simulink model "FOC_algorithm_simulation"  (R2018b)
settings: Solver=VariableStepAuto  StartTime=0.0  StopTime=5  RelTol=1e-3
libraries: simulink x1
settings Model: Creator=杨天山  LastModifiedBy=杨天山

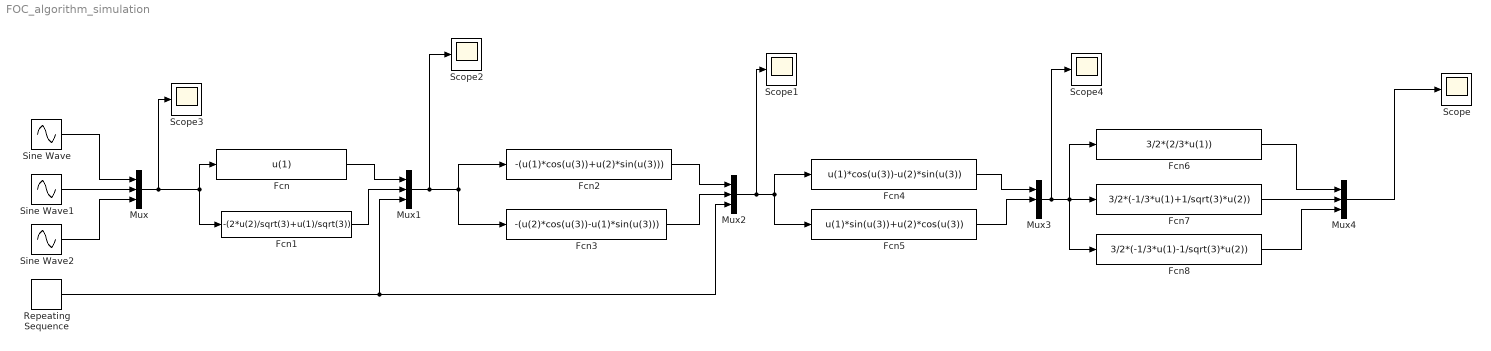
== system FOC_algorithm_simulation ==
  Fcn : Fcn  Expr=u(1)
  Fcn1 : Fcn  Expr=-(2*u(2)/sqrt(3)+u(1)/sqrt(3))
  Fcn2 : Fcn  Expr=-(u(1)*cos(u(3))+u(2)*sin(u(3)))
  Fcn3 : Fcn  Expr=-(u(2)*cos(u(3))-u(1)*sin(u(3)))
  Fcn4 : Fcn  Expr=u(1)*cos(u(3))-u(2)*sin(u(3))
  Fcn5 : Fcn  Expr=u(1)*sin(u(3))+u(2)*cos(u(3))
  Fcn6 : Fcn  Expr=3/2*(2/3*u(1))
  Fcn7 : Fcn  Expr=3/2*(-1/3*u(1)+1/sqrt(3)*u(2))
  Fcn8 : Fcn  Expr=3/2*(-1/3*u(1)-1/sqrt(3)*u(2))
  Mux{,1..4} (5 alike) : Mux  Inputs=3
  Repeating Sequence : simulink/Sources/Repeating Sequence  rep_seq_t=[0 0.1]  rep_seq_y=[0 2*pi]
  Scope{,1..4} (5 alike) : Scope
  Sine Wave : Sin  Frequency=20*pi  SampleTime=0
  Sine Wave1 : Sin  Frequency=20*pi  Phase=2*pi/3  SampleTime=0
  Sine Wave2 : Sin  Frequency=20*pi  Phase=4*pi/3  SampleTime=0
  wires:
  Sine Wave/1 -> Mux/1
  Sine Wave1/1 -> Mux/2
  Sine Wave2/1 -> Mux/3
  Mux/1 -> Scope3/1, Fcn1/1, Fcn/1
  Fcn/1 -> Mux1/1
  Fcn1/1 -> Mux1/2
  Mux1/1 -> Scope2/1, Fcn3/1, Fcn2/1
  Fcn2/1 -> Mux2/1
  Fcn3/1 -> Mux2/2
  Mux2/1 -> Scope1/1, Fcn5/1, Fcn4/1
  Fcn4/1 -> Mux3/1
  Fcn5/1 -> Mux3/2
  Repeating Sequence/1 -> Mux1/3, Mux2/3
  Mux3/1 -> Scope4/1, Fcn8/1, Fcn7/1, Fcn6/1
  Fcn6/1 -> Mux4/1
  Fcn7/1 -> Mux4/2
  Fcn8/1 -> Mux4/3
  Mux4/1 -> Scope/1
